simulink model "gm_flyback_pid"  (R2021b)
settings: Solver=FixedStepDiscrete  StartTime=0.0  StopTime=100e-3  RelTol=1e-3
undefined symbols (not defined in the file or in its folder): DiscIntNeverNeededParam
Description:
  | Symmetric FIR Filter
  | This example shows how to use HDL Coder(TM) to check, generate,
  | and verify HDL for a fixed-point symmetric FIR filter.
settings Model: Creator=The MathWorks, Inc.  LastModifiedBy=Marco Milanesi
settings SolverCC: AlgebraicLoopSolver=TrustRegion  AutoInsertRateTranBlk=on
settings DataIOCC: LimitDataPoints=on  SaveFormat=Array  SaveOutput=off  SignalLogging=off  SaveTime=off  ReturnWorkspaceOutputs=off  SignalLoggingName=logsOut
settings OptimizationCC: BlockReduction=off  BooleanDataType=off  ConditionallyExecuteInputs=off  DefaultParameterBehavior=Inlined  InheritOutputTypeSmallerThanSingle=on  InlineInvariantSignals=on  ExpressionDepthLimit=2147483647  InitFltsAndDblsToZero=on  LifeSpan=inf  BufferReusableBoundary=off
settings DebuggingCC: AlgebraicLoopMsg=error  SaveWithParameterizedLinksMsg=none  UnderspecifiedInitializationDetection=Classic  MergeDetectMultiDrivingBlocksExec=none  CheckExecutionContextPreStartOutputMsg=on  SignalResolutionControl=TryResolveAllWithWarning  InheritedTsInSrcMsg=none  MultiTaskDSMMsg=warning  MultiTaskCondExecSysMsg=none  SingleTaskRateTransMsg=error  IntegerOverflowMsg=none  ParameterPrecisionLossMsg=none  FcnCallInpInsideContextMsg=warning  BusObjectLabelMismatch=none  StateNameClashWarn=warning  SFUnexpectedBacktrackingDiag=warning  SFNoUnconditionalDefaultTransitionDiag=warning  SFExecutionAtInitializationDiag=none  SFMachineParentedDataDiag=warning  IntegerSaturationMsg=none  ArithmeticOperatorsInVariantConditions=warning
settings HardwareCC: ProdBitPerPointer=32  ProdBitPerSizeT=32  ProdBitPerPtrDiffT=32  ProdLargestAtomicFloat=None  ProdIntDivRoundTo=Undefined  ProdEndianess=Unspecified  ProdWordSize=32  ProdHWDeviceType=ASIC/FPGA  TargetUnknown=on  ProdEqTarget=off
settings ModelReferenceCC: PropagateSignalLabelsOutOfModel=off
settings SFSimCC: SimUseLocalCustomCode=off  CustomCodeUndefinedFunction=UseInterfaceOnly
settings RTWCC: RTWUseLocalCustomCode=off
settings CodeAppCC: StateflowObjectComments=on
settings GRTTargetCC: TargetFcnLib=ansi_tfl_tmw.mat  TargetLangStandard=C89/C90 (ANSI)  CombineOutputUpdateFcns=off  GRTInterface=on
settings ConfigComp: CovMetricSettings=dw  CovSaveCumulativeToWorkspaceVar=on  CovSaveSingleToWorkspaceVar=on  CovExternalEMLEnable=off

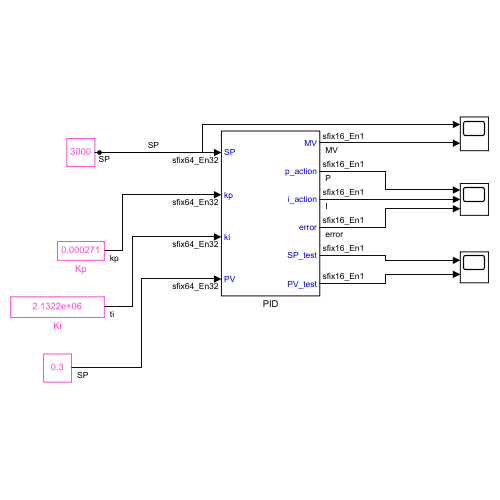
[thumbnail: Simulink's stored preview of the top-level diagram]
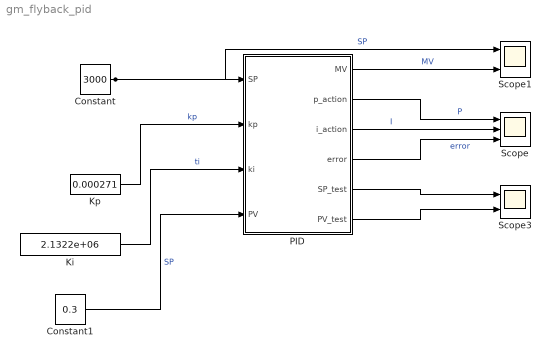
== system gm_flyback_pid ==
  Constant : Constant  Value=3000  OutDataTypeStr=fixdt(1,64,32)
  Constant1 : Constant  Value=0.3  OutDataTypeStr=fixdt(1,64,32)
  Ki : Constant  Value=2.1322e+06  OutDataTypeStr=fixdt(1,64,32)
  Kp : Constant  Value=0.000271  OutDataTypeStr=fixdt(1,64,32)
  PID : Subsystem
  Scope : Scope  NumInputPorts=3
  Scope1 : Scope  NumInputPorts=2
  Scope3 : Scope  NumInputPorts=2
  wires:
  PID/6(PV_test) -> Scope3/2
  PID/5(SP_test) -> Scope3/1
  Constant1/1 -> PID/4(PV)  "SP"
  PID/3(i_action) -> Scope/2  "I"
  PID/1(MV) -> Scope1/2  "MV"
  PID/4(error) -> Scope/3  "error"
  PID/2(p_action) -> Scope/1  "P"
  Constant/1 -> PID/1(SP), Scope1/1  "SP"
  Ki/1 -> PID/3(ki)  "ti"
  Kp/1 -> PID/2(kp)  "kp"

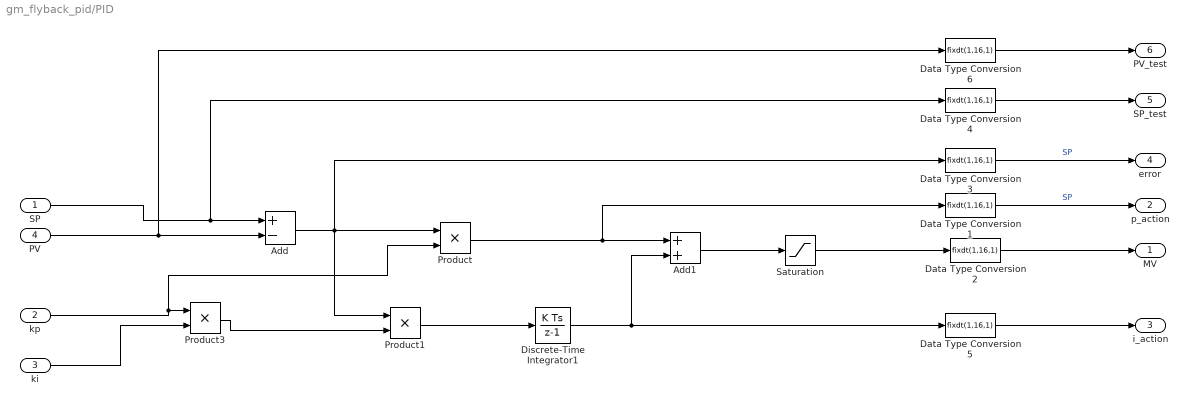
== system gm_flyback_pid/PID ==
  SP : Inport  OutDataTypeStr=fixdt(1,64,32)  SampleTime=1e-3
  kp : Inport  Port=2  OutDataTypeStr=fixdt(1,64,32)  SampleTime=1e-3
  ki : Inport  Port=3  OutDataTypeStr=fixdt(1,64,32)  SampleTime=1e-3
  PV : Inport  Port=4  OutDataTypeStr=fixdt(1,64,32)  SampleTime=1e-3
  Add : Sum  Inputs=+-  AccumDataTypeStr=fixdt(1,64,32)  OutDataTypeStr=fixdt(1,64,32)
  Add1 : Sum  AccumDataTypeStr=fixdt(1,64,32)  OutDataTypeStr=fixdt(1,64,32)
  Data Type Conversion{1..6} (6 alike) : DataTypeConversion  OutDataTypeStr=fixdt(1,16,1)
  Discrete-Time Integrator1 : DiscreteIntegrator  SampleTime=1e-3  OutDataTypeStr=fixdt(1,64,32)  ICPrevOutput=DiscIntNeverNeededParam  ICPrevScaledInput=DiscIntNeverNeededParam
  Product : Product  OutDataTypeStr=fixdt(1,64,32)
  Product1 : Product  OutDataTypeStr=fixdt(1,64,32)
  Product3 : Product  OutDataTypeStr=fixdt(1,64,32)
  Saturation : Saturate  UpperLimit=255  LowerLimit=0  OutDataTypeStr=fixdt(1,64,32)
  MV : Outport  OutDataTypeStr=fixdt(1,16,1)  SampleTime=1e-3  VectorParamsAs1DForOutWhenUnconnected=off
  p_action : Outport  Port=2  OutDataTypeStr=fixdt(1,16,1)  SampleTime=1e-3  VectorParamsAs1DForOutWhenUnconnected=off
  i_action : Outport  Port=3  OutDataTypeStr=fixdt(1,16,1)  SampleTime=1e-3  VectorParamsAs1DForOutWhenUnconnected=off
  error : Outport  Port=4  OutDataTypeStr=fixdt(1,16,1)  SampleTime=1e-3  VectorParamsAs1DForOutWhenUnconnected=off
  SP_test : Outport  Port=5  OutDataTypeStr=fixdt(1,16,1)  SampleTime=1e-3  VectorParamsAs1DForOutWhenUnconnected=off
  PV_test : Outport  Port=6  OutDataTypeStr=fixdt(1,16,1)  SampleTime=1e-3  VectorParamsAs1DForOutWhenUnconnected=off
  wires:
  Data Type Conversion6/1 -> PV_test/1
  SP/1 -> Add/1, Data Type Conversion4/1
  Data Type Conversion4/1 -> SP_test/1
  Data Type Conversion2/1 -> MV/1
  PV/1 -> Add/2, Data Type Conversion6/1
  Saturation/1 -> Data Type Conversion2/1
  Data Type Conversion5/1 -> i_action/1
  Data Type Conversion3/1 -> error/1  "SP"
  Data Type Conversion1/1 -> p_action/1  "SP"
  Discrete-Time Integrator1/1 -> Add1/2, Data Type Conversion5/1
  Product/1 -> Add1/1, Data Type Conversion1/1
  Add/1 -> Product1/1, Product/1, Data Type Conversion3/1
  Product3/1 -> Product1/2
  ki/1 -> Product3/2
  Product1/1 -> Discrete-Time Integrator1/1
  Add1/1 -> Saturation/1
  kp/1 -> Product3/1, Product/2
